simulink model "controlador_trolley"  (R2023b)
settings: Solver=VariableStepAuto  StartTime=0.0  StopTime=10.0  RelTol=1e-3
undefined symbols (not defined in the file): at_max, Ki_v, Kp_v, Ts2, vt_max, xt_0
libraries: simulink x2
settings Model: Creator=Nahuel  LastModifiedBy=Nahuel

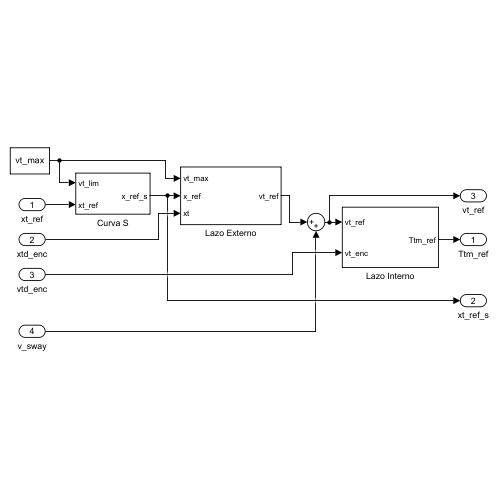
[thumbnail: Simulink's stored preview of the top-level diagram]
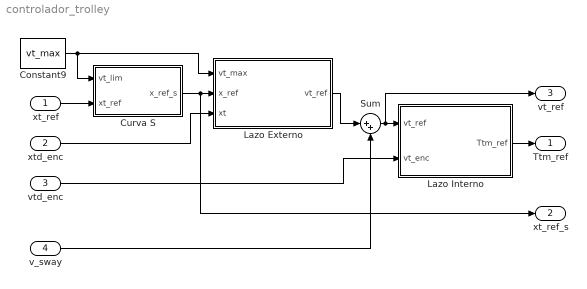
== system controlador_trolley ==
  xt_ref : Inport
  xtd_enc : Inport  Port=2
  vtd_enc : Inport  Port=3
  v_sway : Inport  Port=4
  Constant9 : Constant  Value=vt_max
  Curva S : Subsystem
  Lazo Externo : Subsystem
  Lazo Interno : Subsystem
  Sum : Sum  Inputs=|++
  Ttm_ref : Outport
  xt_ref_s : Outport  Port=2
  vt_ref : Outport  Port=3
  wires:
  Curva S/1(x_ref_s) -> xt_ref_s/1, Lazo Externo/2(x_ref)
  Lazo Interno/1(Ttm_ref) -> Ttm_ref/1
  xt_ref/1 -> Curva S/2(xt_ref)
  Constant9/1 -> Curva S/1(vt_lim), Lazo Externo/1(vt_max)
  Lazo Externo/1(vt_ref) -> Sum/1
  vtd_enc/1 -> Lazo Interno/2(vt_enc)
  xtd_enc/1 -> Lazo Externo/3(xt)
  Sum/1 -> vt_ref/1, Lazo Interno/1(vt_ref)
  v_sway/1 -> Sum/2

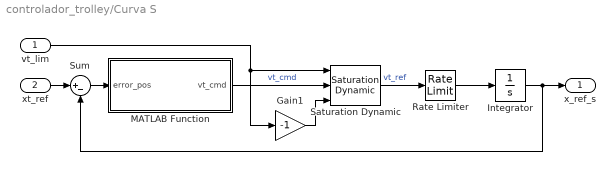
== system controlador_trolley/Curva S ==
  vt_lim : Inport
  xt_ref : Inport  Port=2
  Gain1 : Gain  Gain=-1
  Integrator : Integrator  InitialCondition=xt_0
  MATLAB Function : MATLAB Function  TreatAsAtomicUnit=on
  Rate Limiter : RateLimiter  RisingSlewLimit=at_max  FallingSlewLimit=-at_max  SampleTimeMode=inherited
  Saturation Dynamic : simulink/Discontinuities/Saturation Dynamic  OutMin=[]  OutMax=[]  OutDataTypeStr=Inherit: Same as second input  OutDataType=fixdt(1, 16)  OutScaling=2^-10  DoSatur=off
  Sum : Sum  Inputs=|+-
  x_ref_s : Outport
  wires:
  MATLAB Function/1(vt_cmd) -> Saturation Dynamic/2  "vt_cmd"
  Integrator/1 -> Sum/2, x_ref_s/1
  Rate Limiter/1 -> Integrator/1
  Sum/1 -> MATLAB Function/1(error_pos)
  vt_lim/1 -> Gain1/1, Saturation Dynamic/1
  Gain1/1 -> Saturation Dynamic/3
  Saturation Dynamic/1 -> Rate Limiter/1  "vt_ref"
  xt_ref/1 -> Sum/1

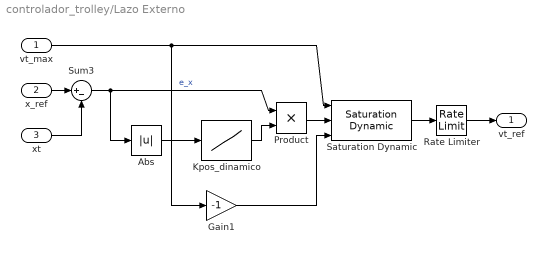
== system controlador_trolley/Lazo Externo ==
  vt_max : Inport
  x_ref : Inport  Port=2
  xt : Inport  Port=3
  Abs : Abs  SaturateOnIntegerOverflow=off
  Gain1 : Gain  Gain=-1
  Kpos_dinamico : Lookup_n-D  NumberOfTableDimensions=1  BreakpointsForDimension1=[0.5;2;5;10;30;50]  Table=[0.25;0.5;0.6;0.8;1;3]  InternalRulePriority=Speed  RndMeth=Simplest
  Product : Product
  Rate Limiter : RateLimiter  RisingSlewLimit=at_max  FallingSlewLimit=-at_max  SampleTimeMode=inherited
  Saturation Dynamic : simulink/Discontinuities/Saturation Dynamic  OutMin=[]  OutMax=[]  OutDataTypeStr=Inherit: Same as second input  OutDataType=fixdt(1, 16)  OutScaling=2^-10  DoSatur=off
  Sum3 : Sum  Inputs=|+-
  vt_ref : Outport
  wires:
  Saturation Dynamic/1 -> Rate Limiter/1
  xt/1 -> Sum3/2
  vt_max/1 -> Gain1/1, Saturation Dynamic/1
  x_ref/1 -> Sum3/1
  Gain1/1 -> Saturation Dynamic/3
  Sum3/1 -> Abs/1, Product/1  "e_x"
  Rate Limiter/1 -> vt_ref/1
  Abs/1 -> Kpos_dinamico/1
  Kpos_dinamico/1 -> Product/2
  Product/1 -> Saturation Dynamic/2

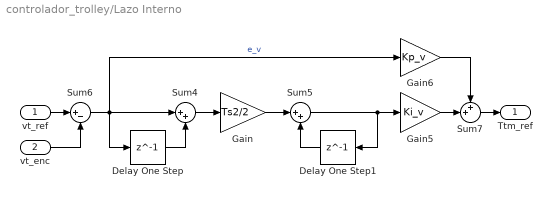
== system controlador_trolley/Lazo Interno ==
  vt_ref : Inport
  vt_enc : Inport  Port=2
  Delay One Step : Delay  DelayLength=1
  Delay One Step1 : Delay  DelayLength=1
  Gain : Gain  Gain=Ts2/2
  Gain5 : Gain  Gain=Ki_v
  Gain6 : Gain  Gain=Kp_v
  Sum4 : Sum  Inputs=|++
  Sum5 : Sum  Inputs=|++
  Sum6 : Sum  Inputs=|+-
  Sum7 : Sum  Inputs=++|
  Ttm_ref : Outport
  wires:
  Sum6/1 -> Gain6/1, Sum4/1, Delay One Step/1  "e_v"
  Delay One Step/1 -> Sum4/2
  Sum5/1 -> Gain5/1, Delay One Step1/1
  Sum7/1 -> Ttm_ref/1
  Gain/1 -> Sum5/1
  Gain5/1 -> Sum7/2
  Delay One Step1/1 -> Sum5/2
  vt_ref/1 -> Sum6/1
  Gain6/1 -> Sum7/1
  Sum4/1 -> Gain/1
  vt_enc/1 -> Sum6/2

== matlab function controlador_trolley/Curva S/MATLAB Function ==
  data: error_pos input; vt_cmd output; at_max parameter
function vt_cmd = Frenado_OptimoT(error_pos, at_max)
    % Parámetro de suavizado (región lineal)
    d_tol = 0.1; % 10 cm de tolerancia donde se vuelve lineal
    
    if abs(error_pos) > d_tol
        % ZONA PARABÓLICA (Frenado Óptimo)
        % Lejos del objetivo, usamos la raíz cuadrada
        vh_brakes = sqrt(2 * at_max * abs(error_pos));
        vt_cmd = vh_brakes * sign(error_pos);
    else
        % ZONA LINEAL (Aterrizaje Suave)
        % Cerca del cero, usamos una ganancia fija para evitar pendiente infinita.
        vh_limit_tol = sqrt(2 * at_max * d_tol); % Velocidad en el borde de la zona
        gain_linear = vh_limit_tol / d_tol;      % Pendiente equivalente        
        vt_cmd = gain_linear * error_pos;
    end
end
